simulink model "Auton_SPF_debug"  (R2023b)
settings: Solver=VariableStepAuto  StartTime=0.0  StopTime=50  MaxStep=t_sample  RelTol=1e-3
undefined symbols (not defined in the file): All_Num_Poses, All_Paths, FloorDistance, t_sample
libraries: simulink x6
settings Model: PauseTimes=10  Creator=ander  LastModifiedBy=ander

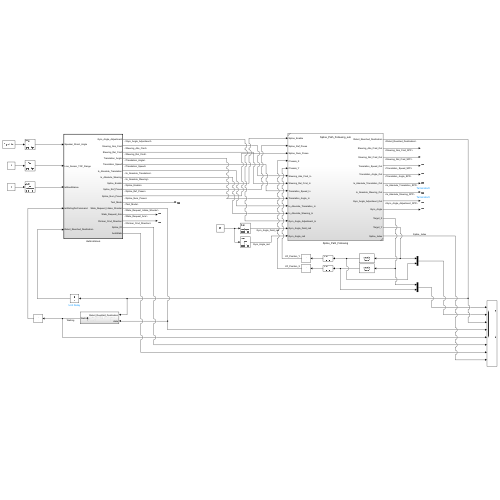
[thumbnail: Simulink's stored preview of the top-level diagram]
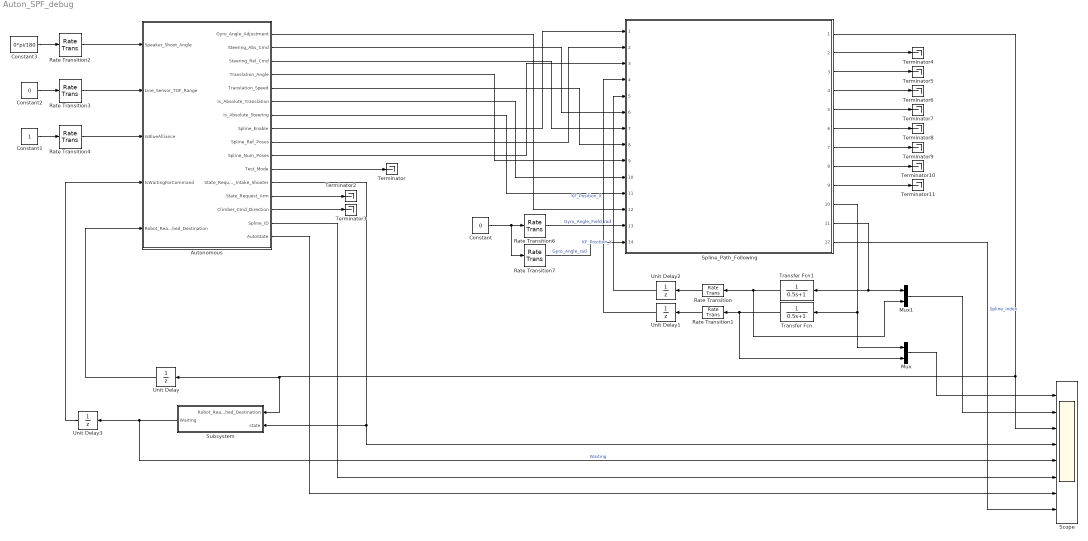
== system Auton_SPF_debug ==
  Autonomous : Subsystem  TreatAsAtomicUnit=on
  Constant : Constant  Value=0
  Constant1 : Constant  OutDataTypeStr=boolean
  Constant2 : Constant  Value=0
  Constant3 : Constant  Value=0*pi/180
  Mux : Mux  Inputs=2
  Mux1 : Mux  Inputs=2
  Rate Transition{,1..4,6..7} (7 alike) : RateTransition  OutPortSampleTime=t_sample
  Scope : Scope  NumInputPorts=8
  Spline_Path_Following : Subsystem  ReferencedSubsystem=Spline_Path_Following_sub
  Subsystem : Subsystem
  Terminator{,2..11} (11 alike) : Terminator
  Transfer Fcn : TransferFcn  Denominator=[0.5 1]
  Transfer Fcn1 : TransferFcn  Denominator=[0.5 1]
  Unit Delay{,1..3} (4 alike) : UnitDelay  SampleTime=-1  HasFrameUpgradeWarning=on
  wires:
  Autonomous/8(Spline_Enable) -> Spline_Path_Following/1
  Autonomous/9(Spline_Ref_Poses) -> Spline_Path_Following/2
  Autonomous/10(Spline_Num_Poses) -> Spline_Path_Following/3
  Autonomous/11(Test_Mode) -> Terminator/1
  Autonomous/13(State_Request_Arm) -> Terminator2/1
  Autonomous/14(Climber_Cmd_Direction) -> Terminator3/1
  Autonomous/7(Is_Absolute_Steering) -> Spline_Path_Following/11
  Autonomous/6(Is_Absolute_Translation) -> Spline_Path_Following/10
  Autonomous/5(Translation_Speed) -> Spline_Path_Following/8
  Autonomous/4(Translation_Angle) -> Spline_Path_Following/9
  Autonomous/3(Steering_Rel_Cmd) -> Spline_Path_Following/7
  Autonomous/2(Steering_Abs_Cmd) -> Spline_Path_Following/6
  Autonomous/1(Gyro_Angle_Adjustment) -> Spline_Path_Following/12
  Spline_Path_Following/2 -> Terminator4/1
  Spline_Path_Following/3 -> Terminator5/1
  Spline_Path_Following/4 -> Terminator6/1
  Spline_Path_Following/5 -> Terminator7/1
  Spline_Path_Following/6 -> Terminator8/1
  Spline_Path_Following/7 -> Terminator9/1
  Spline_Path_Following/8 -> Terminator10/1
  Spline_Path_Following/1 -> Scope/3, Unit Delay/1, Subsystem/1(Robot_Reached_Destination)
  Unit Delay/1 -> Autonomous/5(Robot_Reached_Destination)
  Spline_Path_Following/9 -> Terminator11/1
  Constant/1 -> Rate Transition7/1, Rate Transition6/1
  Constant1/1 -> Rate Transition4/1
  Constant2/1 -> Rate Transition3/1
  Constant3/1 -> Rate Transition2/1
  Spline_Path_Following/10 -> Transfer Fcn/1, Mux/1
  Spline_Path_Following/11 -> Transfer Fcn1/1, Mux1/1
  Transfer Fcn/1 -> Rate Transition1/1, Mux/2
  Transfer Fcn1/1 -> Rate Transition/1, Mux1/2
  Unit Delay1/1 -> Spline_Path_Following/4  "KF_Position_X"
  Unit Delay2/1 -> Spline_Path_Following/5  "KF_Position_Y"
  Rate Transition/1 -> Unit Delay2/1
  Rate Transition1/1 -> Unit Delay1/1
  Rate Transition2/1 -> Autonomous/1(Speaker_Shoot_Angle)
  Rate Transition3/1 -> Autonomous/2(Line_Sensor_TOF_Range)
  Rate Transition4/1 -> Autonomous/3(IsBlueAlliance)
  Rate Transition6/1 -> Spline_Path_Following/13  "Gyro_Angle_Field_rad"
  Rate Transition7/1 -> Spline_Path_Following/14  "Gyro_Angle_rad"
  Mux1/1 -> Scope/2
  Mux/1 -> Scope/1
  Autonomous/12(State_Request_Intake_Shooter) -> Subsystem/2(state), Scope/4
  Subsystem/1(Waiting) -> Unit Delay3/1, Scope/5  "Waiting"
  Unit Delay3/1 -> Autonomous/4(IsWaitingForCommand)
  Autonomous/15(Spline_ID) -> Scope/6
  Autonomous/16(AutoState) -> Scope/7
  Spline_Path_Following/12 -> Scope/8  "Spline_Index"

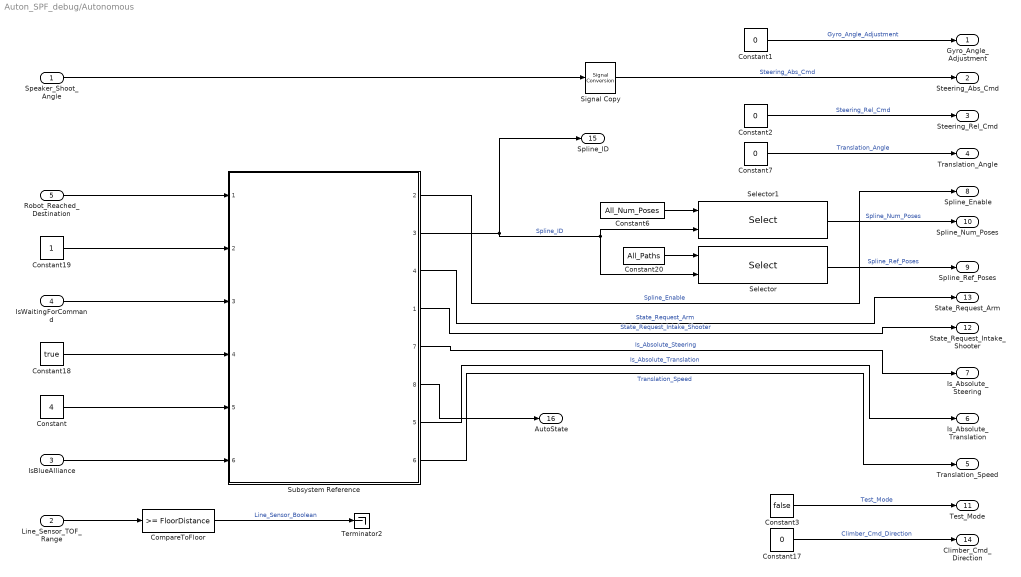
== system Auton_SPF_debug/Autonomous ==
  Speaker_Shoot_Angle : Inport
  Line_Sensor_TOF_Range : Inport  Port=2
  IsBlueAlliance : Inport  Port=3
  IsWaitingForCommand : Inport  Port=4
  Robot_Reached_Destination : Inport  Port=5
  CompareToFloor : simulink/Logic and Bit Operations/Compare To Constant  relop=>=  const=FloorDistance  OutDataTypeStr=boolean
  Constant : Constant  Value=4
  Constant{1..2,7,17} (4 alike) : Constant  Value=0
  Constant18 : Constant  Value=true
  Constant19 : Constant
  Constant20 : Constant  Value=All_Paths
  Constant3 : Constant  Value=false  OutDataTypeStr=boolean
  Constant6 : Constant  Value=All_Num_Poses
  Selector : Selector  NumberOfDimensions=3  InputPortWidth=3  IndexOptions=Select all,Select all,Index vector (port)  Indices=[1 3],1,1  OutputSizes=1,1,1
  Selector1 : Selector  IndexOptions=Index vector (port)  Indices=[1 3]  OutputSizes=1
  Signal Copy : SignalConversion  OverrideOpt=off
  Subsystem Reference : Subsystem  ReferencedSubsystem=State_Interpreter
      settings: PortSchema="{\"entries\":[{\"content\":{\"sides\":[{\"content\":{\"connectorIds\":[\"In1\",\"In2\",\"In3\",\"In4\",\"In5\",\"In6\"]},\"type\":\"ConnectorPlacement.EquallySpacedRectSide\",\"uuid\":\"c9fc2870-041d-4041-9591-a91dffa515e7\"},{\"content\":{\"connectorIds\":[\"Out2\",\"Out3\",\"Out4\",\"Out1\",\"Out7\",\"Out8\",\"Out5\",\"Out6\"],\"side\":\"RIGHT\"},\"type\":\"ConnectorPlacement.EquallySpacedRectSide\",\"uuid\":\"67f8b5c0-38ed-481c-98c9-e8ea4065379a\"},{\"content\":{\"side\":\"TOP\"},\"type\":\"ConnectorPlacement.EquallySpacedRectSide\",\"uuid\":\"331639ac-7071-41dd-8ba3-33fcd3a0d7a0\"}]},\"type\":\"ConnectorPlacement.EquallySpacedConnector\",\"uuid\":\"7f55b551-6349-4f03-a087-ee2e2790c332\"}],\"packageUris\":[\"http://schema.mathworks.com/mf0/Connector/R2020b\"],\"version\":\"1.0\"}"
  Terminator2 : Terminator
  Gyro_Angle_Adjustment : Outport
  Steering_Abs_Cmd : Outport  Port=2
  Steering_Rel_Cmd : Outport  Port=3
  Translation_Angle : Outport  Port=4
  Translation_Speed : Outport  Port=5
  Is_Absolute_Translation : Outport  Port=6
  Is_Absolute_Steering : Outport  Port=7
  Spline_Enable : Outport  Port=8
  Spline_Ref_Poses : Outport  Port=9
  Spline_Num_Poses : Outport  Port=10
  Test_Mode : Outport  Port=11
  State_Request_Intake_Shooter : Outport  Port=12
  State_Request_Arm : Outport  Port=13
  Climber_Cmd_Direction : Outport  Port=14
  Spline_ID : Outport  Port=15
  AutoState : Outport  Port=16
  wires:
  IsBlueAlliance/1 -> Subsystem Reference/6
  Constant/1 -> Subsystem Reference/5
  Constant18/1 -> Subsystem Reference/4
  IsWaitingForCommand/1 -> Subsystem Reference/3
  Signal Copy/1 -> Steering_Abs_Cmd/1  "Steering_Abs_Cmd"
  Subsystem Reference/2 -> Spline_Enable/1  "Spline_Enable"
  Constant20/1 -> Selector/1
  Robot_Reached_Destination/1 -> Subsystem Reference/1
  Constant19/1 -> Subsystem Reference/2
  Constant17/1 -> Climber_Cmd_Direction/1  "Climber_Cmd_Direction"
  Line_Sensor_TOF_Range/1 -> CompareToFloor/1
  CompareToFloor/1 -> Terminator2/1  "Line_Sensor_Boolean"
  Subsystem Reference/1 -> State_Request_Intake_Shooter/1  "State_Request_Intake_Shooter"
  Subsystem Reference/4 -> State_Request_Arm/1  "State_Request_Arm"
  Constant3/1 -> Test_Mode/1  "Test_Mode"
  Subsystem Reference/7 -> Is_Absolute_Steering/1  "Is_Absolute_Steering"
  Subsystem Reference/3 -> Selector1/2, Selector/2, Spline_ID/1  "Spline_ID"
  Subsystem Reference/6 -> Translation_Speed/1  "Translation_Speed"
  Constant7/1 -> Translation_Angle/1  "Translation_Angle"
  Selector1/1 -> Spline_Num_Poses/1  "Spline_Num_Poses"
  Selector/1 -> Spline_Ref_Poses/1  "Spline_Ref_Poses"
  Constant1/1 -> Gyro_Angle_Adjustment/1  "Gyro_Angle_Adjustment"
  Speaker_Shoot_Angle/1 -> Signal Copy/1
  Constant2/1 -> Steering_Rel_Cmd/1  "Steering_Rel_Cmd"
  Subsystem Reference/5 -> Is_Absolute_Translation/1  "Is_Absolute_Translation"
  Constant6/1 -> Selector1/1
  Subsystem Reference/8 -> AutoState/1

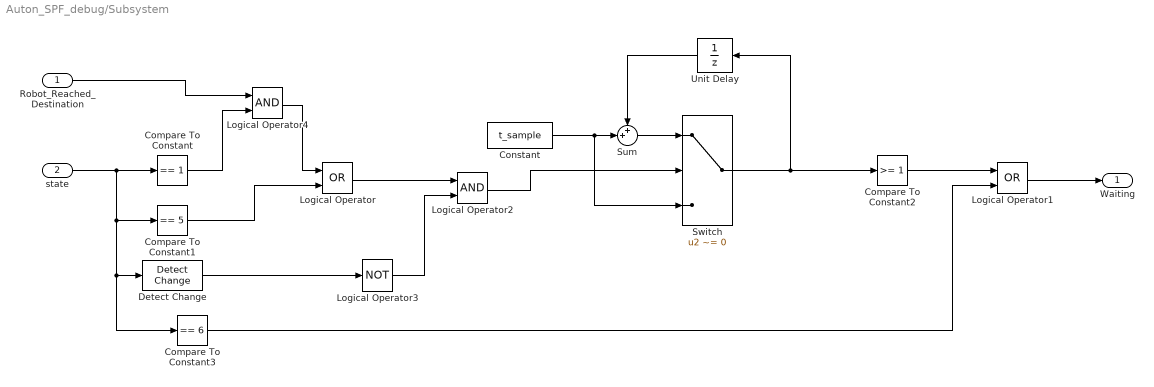
== system Auton_SPF_debug/Subsystem ==
  Robot_Reached_Destination : Inport
  state : Inport  Port=2
  Compare To Constant : simulink/Logic and Bit Operations/Compare To Constant  relop===  const=1  OutDataTypeStr=boolean
  Compare To Constant1 : simulink/Logic and Bit Operations/Compare To Constant  relop===  const=5  OutDataTypeStr=boolean
  Compare To Constant2 : simulink/Logic and Bit Operations/Compare To Constant  relop=>=  const=1  OutDataTypeStr=boolean
  Compare To Constant3 : simulink/Logic and Bit Operations/Compare To Constant  relop===  const=6  OutDataTypeStr=boolean
  Constant : Constant  Value=t_sample
  Detect Change : simulink/Logic and Bit Operations/Detect Change  vinit=0  OutDataTypeStr=boolean
  Logical Operator : Logic  Operator=OR  AllPortsSameDT=off  OutDataTypeStr=boolean
  Logical Operator1 : Logic  Operator=OR  AllPortsSameDT=off  OutDataTypeStr=boolean
  Logical Operator2 : Logic  AllPortsSameDT=off  OutDataTypeStr=boolean
  Logical Operator3 : Logic  Operator=NOT  AllPortsSameDT=off  OutDataTypeStr=boolean
  Logical Operator4 : Logic  AllPortsSameDT=off  OutDataTypeStr=boolean
  Sum : Sum  Inputs=++|
  Switch : Switch  Criteria=u2 ~= 0  SaturateOnIntegerOverflow=off  InputSameDT=off
  Unit Delay : UnitDelay  SampleTime=-1  HasFrameUpgradeWarning=on
  Waiting : Outport
  wires:
  state/1 -> Detect Change/1, Compare To Constant3/1, Compare To Constant1/1, Compare To Constant/1
  Constant/1 -> Switch/3, Sum/2
  Sum/1 -> Switch/1
  Switch/1 -> Compare To Constant2/1, Unit Delay/1
  Unit Delay/1 -> Sum/1
  Compare To Constant2/1 -> Logical Operator1/1
  Compare To Constant3/1 -> Logical Operator1/2
  Logical Operator1/1 -> Waiting/1
  Logical Operator3/1 -> Logical Operator2/2
  Detect Change/1 -> Logical Operator3/1
  Logical Operator2/1 -> Switch/2
  Compare To Constant/1 -> Logical Operator4/2
  Logical Operator/1 -> Logical Operator2/1
  Robot_Reached_Destination/1 -> Logical Operator4/1
  Logical Operator4/1 -> Logical Operator/1
  Compare To Constant1/1 -> Logical Operator/2
